simulink model "ballbeam_sim"  (R2015a)
settings: Solver=ode45  StartTime=0.0  StopTime=200  RelTol=1e-3
InitFcn:
  | param
undefined symbols (not defined in the file or in its folder): ballbeam_SSctrl, drawBallBeam, P
settings Model: Creator=beard  LastModifiedBy=ecestudent
settings DataIOCC: SignalLoggingSaveFormat=ModelDataLogs
settings OptimizationCC: ExpressionDepthLimit=2147483647  InitFltsAndDblsToZero=on
settings DebuggingCC: UnderspecifiedInitializationDetection=Classic  MergeDetectMultiDrivingBlocksExec=none  SolverPrmCheckMsg=warning  FcnCallInpInsideContextMsg=UseLocalSettings  StateNameClashWarn=warning
settings GRTTargetCC: CombineOutputUpdateFcns=off  GRTInterface=on

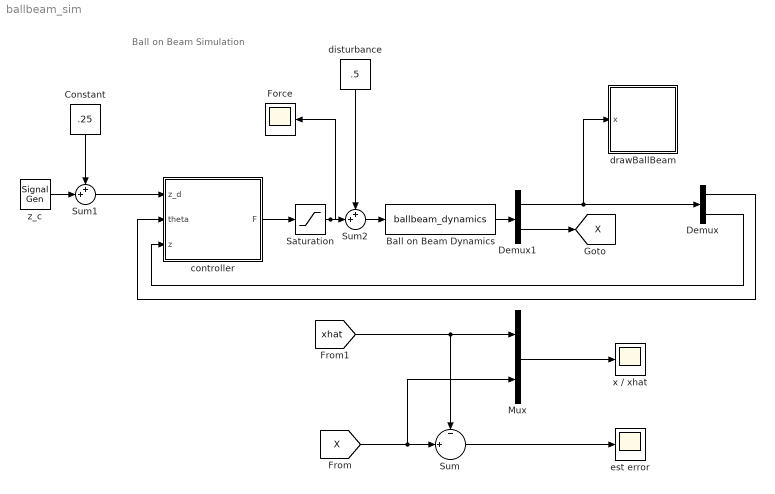
== system ballbeam_sim ==
  note: Ball on Beam Simulation
  Ball on Beam Dynamics : S-Function  FunctionName=ballbeam_dynamics  Parameters=AP
  Constant : Constant  Value=.25
  Demux : Demux  Outputs=2
  Demux1 : Demux  Outputs=[2 4]
  Force : Scope
      settings: YMin=6  YMax=13  SaveName=ScopeData2
  Mux : Mux  Inputs=2
  Saturation : Saturate  UpperLimit=P.Fmax  LowerLimit=-P.Fmax
  Sum : Sum  Inputs=-|+||
  Sum1 : Sum  Inputs=++|
  Sum2 : Sum  Inputs=++|
  controller : Subsystem
  disturbance : Constant  Value=.5
  drawBallBeam : Subsystem
      mask Display: image(imread('tv.jpg'))
  est error : Scope
      settings: TimeRange=200  YMin=-0.5  YMax=0.3  SaveName=ScopeData4
  x / xhat : Scope
      settings: YMin=-0.2  YMax=0.5  SaveName=ScopeData3
  z_c : SignalGenerator  WaveForm=square  Amplitude=.15  Frequency=.02
  tag scope: X=global
  wires:
  z_c/1 -> Sum1/2
  Sum1/1 -> controller/1(z_d)
  Constant/1 -> Sum1/1
  Saturation/1 -> Force/1, Sum2/2
  controller/1(F) -> Saturation/1
  Demux/2 -> controller/3(z)
  Demux/1 -> controller/2(theta)
  Ball on Beam Dynamics/1 -> Demux1/1
  Demux1/1 -> drawBallBeam/1(x), Demux/1
  Demux1/2 -> [X]
  [X] -> Mux/2, Sum/2
  [xhat] -> Sum/1, Mux/1
  Mux/1 -> x / xhat/1
  Sum/1 -> est error/1
  Sum2/1 -> Ball on Beam Dynamics/1
  disturbance/1 -> Sum2/1

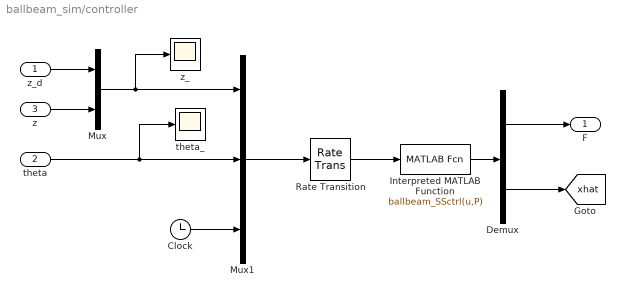
== system ballbeam_sim/controller ==
  z_d : Inport
  theta : Inport  Port=2
  z : Inport  Port=3
  Clock : Clock
  Demux : Demux  Outputs=2
  Interpreted MATLAB Function : MATLABFcn  MATLABFcn=ballbeam_SSctrl(u,P)  OutputDimensions=5
  Mux : Mux  Inputs=2
  Mux1 : Mux  Inputs=3
  Rate Transition : RateTransition  OutPortSampleTime=P.Ts
  theta_ : Scope
      settings: TimeRange=100  YMin=-2  YMax=1.5
  z_ : Scope
      settings: TimeRange=100  YMin=0.025  YMax=0.475
  F : Outport
  tag scope: xhat=global
  wires:
  Mux1/1 -> Rate Transition/1
  Rate Transition/1 -> Interpreted MATLAB Function/1
  theta/1 -> theta_/1, Mux1/2
  z_d/1 -> Mux/1
  z/1 -> Mux/2
  Mux/1 -> z_/1, Mux1/1
  Clock/1 -> Mux1/3
  Interpreted MATLAB Function/1 -> Demux/1
  Demux/1 -> F/1
  Demux/2 -> [xhat]

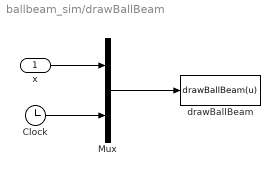
== system ballbeam_sim/drawBallBeam ==
  x : Inport
  Clock : Clock
  Mux : Mux  Inputs=2
  drawBallBeam : MATLABFcn  MATLABFcn=drawBallBeam(u)  OutputDimensions=0  SampleTime=0.1
  wires:
  Mux/1 -> drawBallBeam/1
  x/1 -> Mux/1
  Clock/1 -> Mux/2
